simulink model "untitled"  (Simulink 8.0)
settings: Solver=ode3  StartTime=0.0  StopTime=tf  FixedStep=TS  RelTol=1e-3
libraries: powerlib_extras x1
settings Model: Creator=corsi  LastModifiedBy=corsi

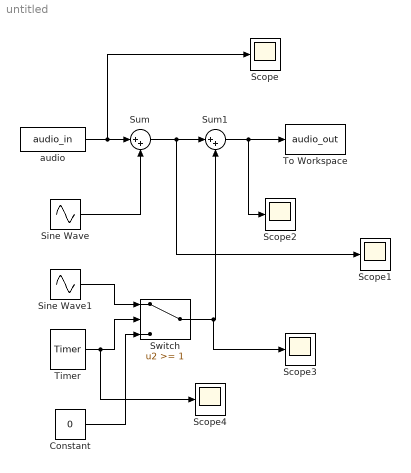
== system untitled ==
  Constant : Constant  Value=0
  Scope{,1..4} (5 alike) : Scope
      Scope settings: YMin=-0.5  YMax=0.3
      Scope2 settings: SaveName=ScopeData2
      Scope3 settings: SaveName=ScopeData3
      Scope4 settings: SaveName=ScopeData4
  Sine Wave : Sin  Amplitude=0.5  Frequency=1000*2*pi
  Sine Wave1 : Sin  Amplitude=0.1  Frequency=5000*2*pi
  Sum : Sum  Inputs=|++
  Sum1 : Sum  Inputs=|++
  Switch : Switch  Threshold=1
  Timer : powerlib_extras/Control  Blocks/Timer  t="[ 0  5 10]"  e="[0  1 0]"
  To Workspace : ToWorkspace  VariableName=audio_out  SampleTime=-1  SaveFormat=Timeseries
  audio : FromWorkspace  VariableName=audio_in
  wires:
  audio/1 -> Sum/1, Scope/1
  Sum/1 -> Scope1/1, Sum1/1
  Sine Wave/1 -> Sum/2
  Sum1/1 -> Scope2/1, To Workspace/1
  Switch/1 -> Scope3/1, Sum1/2
  Timer/1 -> Scope4/1, Switch/2
  Constant/1 -> Switch/3
  Sine Wave1/1 -> Switch/1
